simulink model "brazodosgradospatito"  (R2013a)
settings: Solver=ode23s  StartTime=0.0  StopTime=100  RelTol=1e-3
settings Model: Creator=Daniel  LastModifiedBy=Daniel

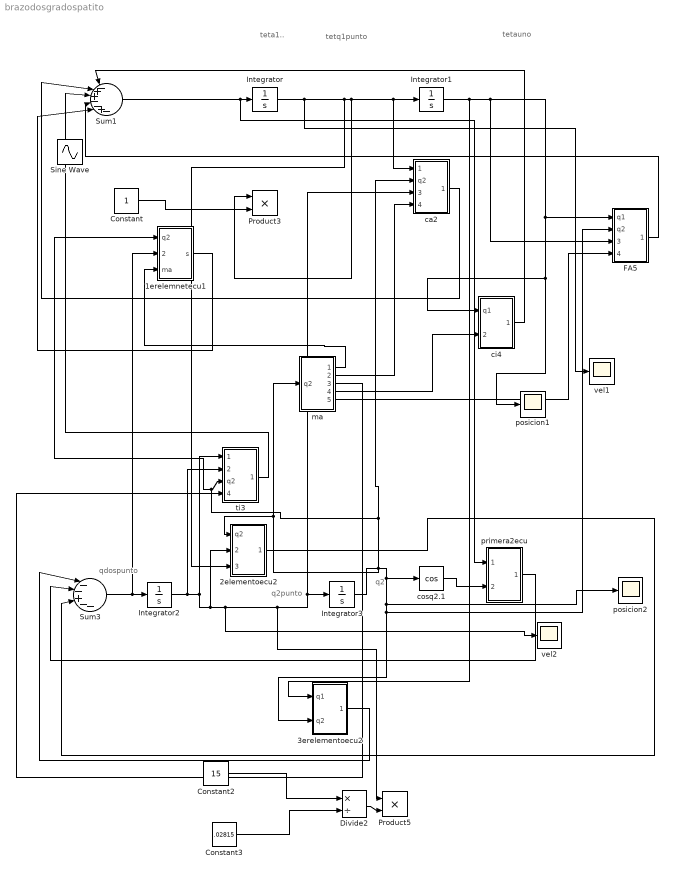
== system brazodosgradospatito ==
  note: q2
  note: q2punto
  note: qdospunto
  note: teta1..
  note: tetauno
  note: tetq1punto
  1erelemnetecu1 : Subsystem
  2elementoecu2 : Subsystem
  3erelementoecu2 : Subsystem
  Constant : Constant
  Constant2 : Constant  Value=15
  Constant3 : Constant  Value=.02815
  Divide2 : Product  Inputs=*/
  FA5 : Subsystem
  Integrator : Integrator
  Integrator1 : Integrator  InitialCondition=pi
  Integrator2 : Integrator
  Integrator3 : Integrator  InitialCondition=pi
  Product3 : Product
  Product5 : Product
  Sine Wave : Sin  SampleTime=0
  Sum1 : Sum  Inputs=|-++--+-
  Sum3 : Sum  Inputs=|--+--
  "ca2 " : Subsystem  VariantControl=Variant1
  ci4 : Subsystem
  cosq2.1 : Trigonometry  Operator=cos
  ma : Subsystem
  posicion1 : Scope
  posicion2 : Scope
  primera2ecu : Subsystem
  ti3 : Subsystem
  vel1 : Scope
      settings: SaveName=mio
  vel2 : Scope
      settings: SaveName=mio1
  wires:
  Integrator1/1 -> 3erelementoecu2/1(q1), FA5/3(q1si), posicion1/1, ci4/1(q1), FA5/1(q1)
  "ca2 "/1(Out1) -> Sum1/2
  FA5/1(out) -> Sum1/4
  ci4/1(Out1) -> Sum1/1
  ti3/1(Out1) -> Sum1/3
  cosq2.1/1 -> primera2ecu/2(cosq2)
  primera2ecu/1(Out1) -> Sum3/2
  2elementoecu2/1(Out1) -> Sum3/3
  Sum3/1 -> Integrator2/1, 1erelemnetecu1/2(q2puntos)
  Integrator3/1 -> ma/1(q2), 2elementoecu2/1(q2), "ca2 "/2(q2), 1erelemnetecu1/1(q2), ti3/3(q2), FA5/2(q2), 3erelementoecu2/2(q2), posicion2/1, cosq2.1/1
  3erelementoecu2/1(Out1) -> Sum3/1
  Integrator/1 -> vel1/1, 2elementoecu2/3(q1.), Product3/1, "ca2 "/1(q1.), Integrator1/1
  Constant2/1 -> Divide2/1
  Integrator2/1 -> ti3/2(q2.), 2elementoecu2/2(q2.), vel2/1, Product5/1, "ca2 "/3(q2.), Integrator3/1, ti3/1(q2.1)
  Constant3/1 -> Divide2/2
  Divide2/1 -> Product5/2
  1erelemnetecu1/1(s) -> Sum1/5
  Sum1/1 -> primera2ecu/1(q1..), Integrator/1
  ma/1(Out1) -> 1erelemnetecu1/3(ma)
  ma/2(Out2) -> "ca2 "/4(ma)
  ma/3(Out3) -> ti3/4(ma)
  ma/4(Out4) -> ci4/2(ma)
  ma/5(Out5) -> FA5/4(ma)
  Constant/1 -> Product3/2

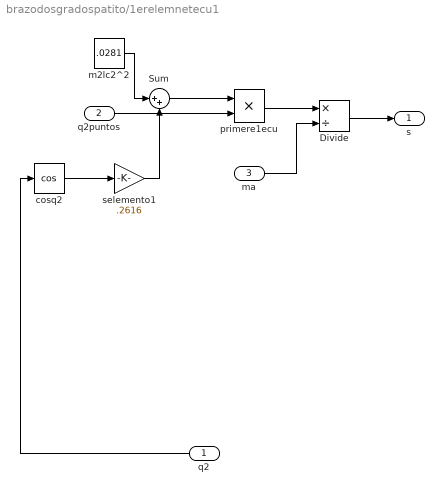
== system brazodosgradospatito/1erelemnetecu1 ==
  q2 : Inport
  q2puntos : Inport  Port=2
  ma : Inport  Port=3
  Divide : Product  Inputs=*/
  Sum : Sum  Inputs=|++
  cosq2 : Trigonometry  Operator=cos
  m2lc2^2 : Constant  Value=.0281
  primere1ecu : Product
  "selemento1 " : Gain  Gain=.2616
  s : Outport
  wires:
  m2lc2^2/1 -> Sum/1
  cosq2/1 -> "selemento1 "/1
  "selemento1 "/1 -> Sum/2
  Sum/1 -> primere1ecu/1
  q2/1 -> cosq2/1
  q2puntos/1 -> primere1ecu/2
  primere1ecu/1 -> Divide/1
  ma/1 -> Divide/2
  Divide/1 -> s/1

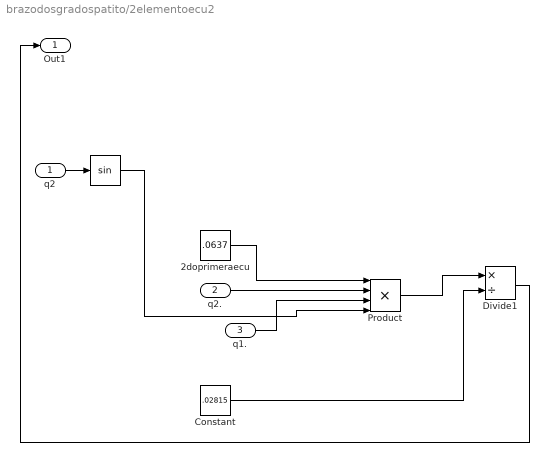
== system brazodosgradospatito/2elementoecu2 ==
  q2 : Inport
  q2. : Inport  Port=2
  q1. : Inport  Port=3
  " " : Trigonometry
  "2doprimeraecu " : Constant  Value=.0637
  Constant : Constant  Value=.02815
  Divide1 : Product  Inputs=*/
  Product : Product  Inputs=4
  Out1 : Outport
  wires:
  q1./1 -> Product/3
  q2./1 -> Product/2
  q2/1 -> " "/1
  " "/1 -> Product/4
  "2doprimeraecu "/1 -> Product/1
  Product/1 -> Divide1/1
  Constant/1 -> Divide1/2
  Divide1/1 -> Out1/1

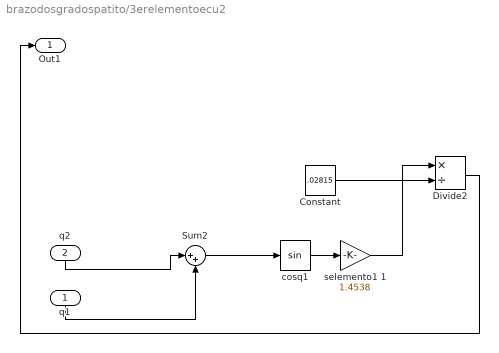
== system brazodosgradospatito/3erelementoecu2 ==
  q1 : Inport
  q2 : Inport  Port=2
  Constant : Constant  Value=.02815
  Divide2 : Product  Inputs=*/
  Sum2 : Sum  Inputs=|++
  cosq1 : Trigonometry
  selemento1 1 : Gain  Gain=1.4538
  Out1 : Outport
  wires:
  Divide2/1 -> Out1/1
  q1/1 -> Sum2/2
  q2/1 -> Sum2/1
  selemento1 1/1 -> Divide2/1
  Sum2/1 -> cosq1/1
  cosq1/1 -> selemento1 1/1
  Constant/1 -> Divide2/2

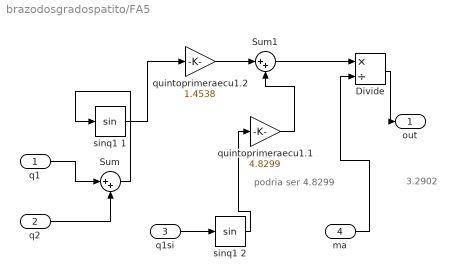
== system brazodosgradospatito/FA5 ==
  note: 3.2902
  note: podria ser 4.8299
  q1 : Inport
  q2 : Inport  Port=2
  q1si : Inport  Port=3
  ma : Inport  Port=4
  Divide : Product  Inputs=*/
  Sum : Sum  Inputs=|++
  Sum1 : Sum  Inputs=|++
  quintoprimeraecu1.1 : Gain  Gain=4.8299  LockScale=on
  quintoprimeraecu1.2 : Gain  Gain=1.4538  LockScale=on
  sinq1 1 : Trigonometry
  sinq1 2 : Trigonometry
  out : Outport
  wires:
  sinq1 1/1 -> quintoprimeraecu1.2/1
  quintoprimeraecu1.2/1 -> Sum1/1
  q1/1 -> Sum/1
  q2/1 -> Sum/2
  Sum/1 -> sinq1 1/1
  q1si/1 -> sinq1 2/1
  sinq1 2/1 -> quintoprimeraecu1.1/1
  quintoprimeraecu1.1/1 -> Sum1/2
  Sum1/1 -> Divide/1
  ma/1 -> Divide/2
  Divide/1 -> out/1

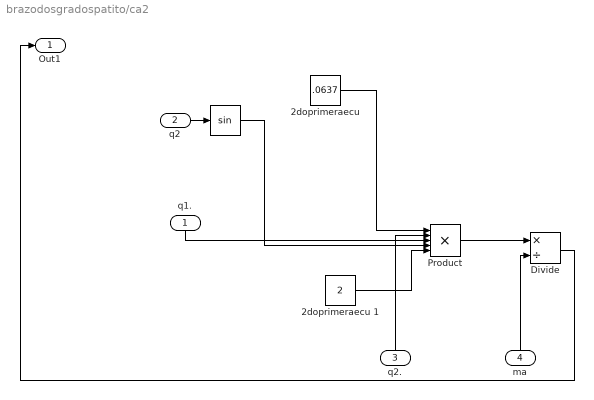
== system brazodosgradospatito/ca2  ==
  q1. : Inport
  q2 : Inport  Port=2
  q2. : Inport  Port=3
  ma : Inport  Port=4
  " " : Trigonometry
  "2doprimeraecu " : Constant  Value=.0637
  2doprimeraecu 1 : Constant  Value=2
  Divide : Product  Inputs=*/
  Product : Product  Inputs=5
  Out1 : Outport
  wires:
  q2/1 -> " "/1
  " "/1 -> Product/4
  q2./1 -> Product/2
  "2doprimeraecu "/1 -> Product/1
  q1./1 -> Product/3
  2doprimeraecu 1/1 -> Product/5
  Product/1 -> Divide/1
  ma/1 -> Divide/2
  Divide/1 -> Out1/1

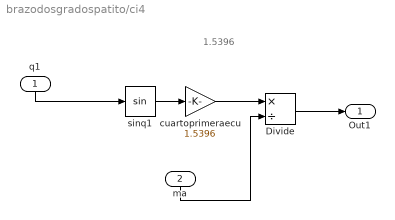
== system brazodosgradospatito/ci4 ==
  note: 1.5396
  q1 : Inport
  ma : Inport  Port=2
  Divide : Product  Inputs=*/
  cuartoprimeraecu : Gain  Gain=1.5396  LockScale=on
  "sinq1 " : Trigonometry
  Out1 : Outport
  wires:
  q1/1 -> "sinq1 "/1
  "sinq1 "/1 -> cuartoprimeraecu/1
  cuartoprimeraecu/1 -> Divide/1
  Divide/1 -> Out1/1
  ma/1 -> Divide/2

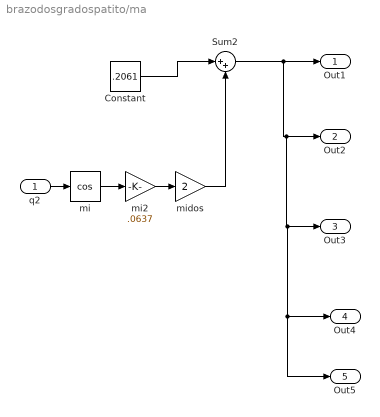
== system brazodosgradospatito/ma ==
  q2 : Inport
  Constant : Constant  Value=.2061
  Sum2 : Sum  Inputs=|++
  mi : Trigonometry  Operator=cos
  "mi2 " : Gain  Gain=.0637
  "midos " : Gain  Gain=2
  Out1 : Outport
  Out2 : Outport  Port=2
  Out3 : Outport  Port=3
  Out4 : Outport  Port=4
  Out5 : Outport  Port=5
  wires:
  "mi2 "/1 -> "midos "/1
  mi/1 -> "mi2 "/1
  Constant/1 -> Sum2/1
  "midos "/1 -> Sum2/2
  q2/1 -> mi/1
  Sum2/1 -> Out5/1, Out4/1, Out3/1, Out2/1, Out1/1

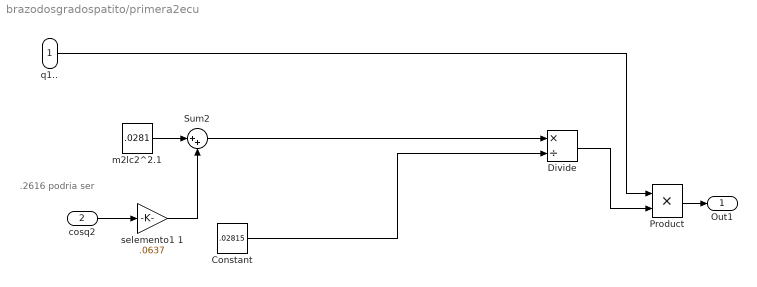
== system brazodosgradospatito/primera2ecu ==
  note: .2616 podria ser
  q1.. : Inport
  cosq2 : Inport  Port=2
  Constant : Constant  Value=.02815
  Divide : Product  Inputs=*/
  Product : Product
  Sum2 : Sum  Inputs=|++
  m2lc2^2.1 : Constant  Value=.0281
  selemento1 1 : Gain  Gain=.0637
  Out1 : Outport
  wires:
  cosq2/1 -> selemento1 1/1
  selemento1 1/1 -> Sum2/2
  m2lc2^2.1/1 -> Sum2/1
  Constant/1 -> Divide/2
  Sum2/1 -> Divide/1
  Product/1 -> Out1/1
  Divide/1 -> Product/2
  q1../1 -> Product/1

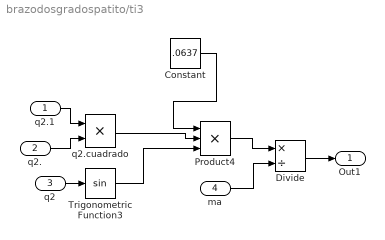
== system brazodosgradospatito/ti3 ==
  q2.1 : Inport
  q2. : Inport  Port=2
  q2 : Inport  Port=3
  ma : Inport  Port=4
  Constant : Constant  Value=.0637
  Divide : Product  Inputs=*/
  Product4 : Product  Inputs=3
  Trigonometric Function3 : Trigonometry
  q2.cuadrado : Product
  Out1 : Outport
  wires:
  q2./1 -> q2.cuadrado/2
  q2.1/1 -> q2.cuadrado/1
  q2/1 -> Trigonometric Function3/1
  q2.cuadrado/1 -> Product4/2
  Trigonometric Function3/1 -> Product4/3
  Constant/1 -> Product4/1
  Product4/1 -> Divide/1
  ma/1 -> Divide/2
  Divide/1 -> Out1/1
